simulink model "GSFR_Individual_Vars"  (R2019b)
settings: Solver=VariableStepAuto  StartTime=0  StopTime=20.0  MaxStep=0.01  RelTol=1e-3
model workspace (MAT data in the model file):
  H = [8 1]
values from neighbouring files (symbols this model uses):
  Pd = -0.1    [Monte_Carlo_GSFR_Ideal_Injection.m]    (also in Pd_and_Injection_Model_Run.m = -0.3; Simulink_Approach_Jesus.m = -0.3; dpt_from_dft_H.m = -0.3)
settings Model: EnablePacing=on  PacingRate=1000  ParameterArgumentNames=H  OrderedModelArguments=off  Creator=ruiva  LastModifiedBy=ruiva

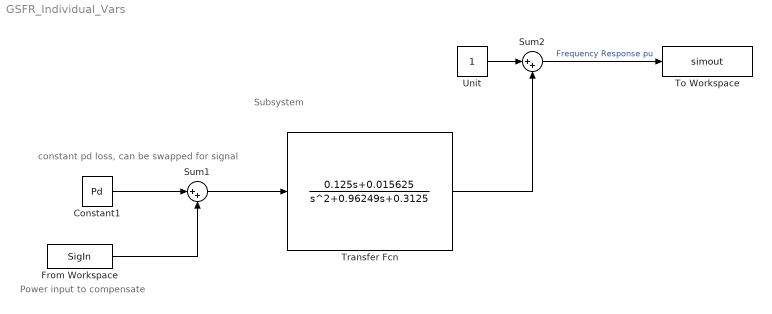
== system GSFR_Individual_Vars ==
  note: Subsystem
  note: Power input to compensate
  note: constant pd loss, can be swapped for signal
  Constant1 : Constant  Value=Pd
  From Workspace : FromWorkspace  VariableName=SigIn  SampleTime=0
  Sum1 : Sum  Inputs=|++
  Sum2 : Sum  Inputs=|++
  To Workspace : ToWorkspace  VariableName=simout  SaveFormat=Timeseries  SampleTime=-1
  Transfer Fcn : TransferFcn  Numerator=[0.125 0.015625]  Denominator=[1 0.96249 0.3125]
  Unit : Constant
  wires:
  Transfer Fcn/1 -> Sum2/2
  Unit/1 -> Sum2/1
  Sum2/1 -> To Workspace/1  "Frequency Response pu"
  From Workspace/1 -> Sum1/2
  Sum1/1 -> Transfer Fcn/1
  Constant1/1 -> Sum1/1
